simulink model "Consigna5_2_1"  (R2024b)
settings: Solver=ode45  StartTime=0.0  StopTime=20  RelTol=1e-3
values from neighbouring files (symbols this model uses):
  A_corrientes = [0 1; -omega_n_corrientes^2 -2*omega_n_corrientes]    [parametros.m]
  A_inversor = [0 1; -omega_n_inversor^2 -2*omega_n_inversor]    [parametros.m]
  A_posicion = [0 1; -omega_n_posicion^2 -2*omega_n_posicion]    [parametros.m]
  A_temp = -1/20    (= -0.05)    [parametros.m]
  alpha_cu = 3.9 *10^-3    (= 0.0039)    [parametros.m]
  B_corrientes = [0; omega_n_corrientes^2]    [parametros.m]
  b_eq = b_m + (1/r^2) * b_l    (= 2.19444444444e-05)    [parametros.m]
  B_inversor = [0; omega_n_inversor^2]    [parametros.m]
  b_l = 0.1    [parametros.m]
  b_m = 1.5 * 10^-5    (= 1.5e-05)    [parametros.m]
  B_posicion = [0; omega_n_posicion^2]    [parametros.m]
  B_temp = 1/20    (= 0.05)    [parametros.m]
  ba = J_eq*n*omega_pos    (= 0.0916527777778)    [parametros.m]
  C_corrientes = [1 0]    [parametros.m]
  C_inversor = [1 0]    [parametros.m]
  C_posicion = [1 0]    [parametros.m]
  C_temp = 1    [parametros.m]
  C_ts = 0.818    [parametros.m]
  g = 9.80665    [parametros.m]
  J_l = (m*l_cm^2 + J_cm) + (m_l * l_l^2)    (= 0.4583)    [parametros.m]
  J_m = 1.4 * 10^-5    (= 1.4e-05)    [parametros.m]
  K_e_int = 3200 ^3    (= 32768000000)    [parametros.m]
  K_e_omega = 3*3200^2    (= 30720000)    [parametros.m]
  K_e_theta = 9600    [parametros.m]
  k_l = m * l_cm + m_l* l_l    (= 1)    [parametros.m]
  Ksa = J_eq*n*(omega_pos^2)    (= 73.3222222222)    [parametros.m]
  Ksia = J_eq*(omega_pos^3)    (= 23463.1111111)    [parametros.m]
  L_d = 6.6 * 10^-3    (= 0.0066)    [parametros.m]
  L_ls = 0.8 * 10^-3    (= 0.0008)    [parametros.m]
  L_q = 5.8 * 10^-3    (= 0.0058)    [parametros.m]
  lambda_m = 0.016    [parametros.m]
  P_p = 3    [parametros.m]
  r = 120    [parametros.m]
  R_s_40 = 1.02    [parametros.m]
  R_ts_amb = 146.7    [parametros.m]
  T_sample = 1/f_sample    (= 4.53514739229e-05)    [parametros.m]
  Temp_s_ref = 20    [parametros.m]
  tm = X(1)    [parametros.m]
  tr = X(2)    [parametros.m]
  w2 = 188.49556    [parametros.m]
  x0_corrientes = [0;0]    [parametros.m]
  x0_inversor = [0;0]    [parametros.m]
  x0_posicion = [0; 0]    [parametros.m]
  x0_temp = 20    [parametros.m]
libraries: simulink x14, dspsigops x6
(part 2 of 4)

== system Consigna5_2_1/Subsystem1/Observador de estado reducido ==
  T_m* : Inport
  theta_m : Inport  Port=2
  Gain : Gain  Gain=1/(J_m+(J_l/r^2))
  Gain1 : Gain  Gain=K_e_theta
  Gain2 : Gain  Gain=K_e_omega
  Integrator : Integrator
  Integrator1 : Integrator
  Sum : Sum  Inputs=|++
  Sum1 : Sum  Inputs=|++
  Sum2 : Sum  Inputs=|-+
  omega_m_obs : Outport
  theta_m_obs : Outport  Port=2
  wires:
  T_m*/1 -> Gain/1
  Gain/1 -> Sum/1
  Sum/1 -> Integrator/1
  Integrator1/1 -> theta_m_obs/1, Sum2/1
  Integrator/1 -> Sum1/1
  Sum1/1 -> omega_m_obs/1, Integrator1/1
  theta_m/1 -> Sum2/2
  Gain1/1 -> Sum1/2
  Sum2/1 -> Gain2/1, Gain1/1
  Gain2/1 -> Sum/2

== system Consigna5_2_1/Subsystem1/Setpoint ==
  q1* : Inport
  Derivative : Derivative
  Gain : Gain  Gain=r
  theta_m* : Outport
  omega_m* : Outport  Port=2
  wires:
  q1*/1 -> Gain/1
  Gain/1 -> Derivative/1, theta_m*/1
  Derivative/1 -> omega_m*/1

== system Consigna5_2_1/Subsystem1/Subsistema físico no lineal ==
  note: Retroalimentación natural del torque gravitacional
  T_per : Inport
  v_as : Inport  Port=2
  v_bs : Inport  Port=3
  v_cs : Inport  Port=4
  Tº_amb : Inport  Port=5
  Gain : Gain  Gain=P_p
  Gain1 : Gain  Gain=1/r
  Gain2 : Gain  Gain=k_l
  Gain3 : Gain  Gain=g
  Mux : Mux  Inputs=3
  Scope : Scope
  Sin : Trigonometry
  Subsistema electromagnético : Subsystem
      settings: PortSchema="{\"entries\":[{\"content\":{\"sides\":[{\"content\":{\"connectorIds\":[\"In1\",\"In2\",\"In3\",\"In4\"]},\"type\":\"ConnectorPlacement.EquallySpacedRectSide\",\"uuid\":\"c9fae60f-a644-4c7d-9a50-e330e891aba8\"},{\"content\":{\"connectorIds\":[\"Out1\",\"Out2\",\"Out3\",\"Out4\"],\"side\":\"RIGHT\"},\"type\":\"ConnectorPlacement.EquallySpacedRectSide\",\"uuid\":\"1bd25713-f5e9-4106-83eb-fb9f8a30d88e\"},{\"content\":{\"connectorIds\":[\"In5\"],\"side\":\"TOP\"},\"type\":\"ConnectorPlacement.EquallySpacedRectSide\",\"uuid\":\"c2f005dd-e04f-426d-b804-ce475aa5422d\"}]},\"type\":\"ConnectorPlacement.EquallySpacedConnector\",\"uuid\":\"9bdc4406-fcef-47cb-a5c0-d4f33f547a91\"}],\"packageUris\":[\"http://schema.mathworks.com/mf0/Connector/R2020b\"],\"version\":\"1.0\"}"
  Subsistema mecánico completo : Subsystem
  Subsistema térmico : Subsystem
  Sum : Sum  Inputs=++|
  TD_PARK : MATLAB Function  TreatAsAtomicUnit=on
  TI_PARK : MATLAB Function  TreatAsAtomicUnit=on
  theta_m : Outport
  T_s : Outport  Port=2
  i_abcs : Outport  Port=3
  omega_m : Outport  Port=4
  T_m : Outport  Port=5
  T_l : Outport  Port=6
  wires:
  Subsistema electromagnético/4(T_m) -> T_m/1, Subsistema mecánico completo/1(T_m)
  Subsistema electromagnético/3(i_0s) -> Subsistema térmico/3(i_0s^r), TI_PARK/3(f0s)
  Subsistema mecánico completo/2(omega_m(t)) -> Subsistema electromagnético/5(omega_m), Scope/1, omega_m/1
  Subsistema electromagnético/1(i_qs^r) -> Subsistema térmico/1(i_qs^r), TI_PARK/1(fqs)
  Subsistema electromagnético/2(i_ds^r) -> Subsistema térmico/2(i_ds^r), TI_PARK/2(fds)
  Sum/1 -> T_l/1, Subsistema mecánico completo/2(T_l)  "T_l"
  TD_PARK/1(fqs) -> Subsistema electromagnético/1(v_qs^r)
  Tº_amb/1 -> Subsistema térmico/4(Tº_amb)
  Mux/1 -> i_abcs/1
  TI_PARK/1(fas) -> Mux/1
  TI_PARK/2(fbs) -> Mux/2
  TI_PARK/3(fcs) -> Mux/3
  v_as/1 -> TD_PARK/1(fas)
  v_cs/1 -> TD_PARK/3(fcs)
  Gain/1 -> TI_PARK/4(theta_r), TD_PARK/4(theta_r)
  v_bs/1 -> TD_PARK/2(fbs)
  Gain1/1 -> Sin/1
  Sin/1 -> Gain3/1
  Gain2/1 -> Sum/1
  T_per/1 -> Sum/2
  TD_PARK/2(fds) -> Subsistema electromagnético/2(v_ds^r)
  TD_PARK/3(f0s) -> Subsistema electromagnético/3(v_0s)
  Subsistema térmico/1(r_s) -> Subsistema electromagnético/4(r_s)
  Subsistema térmico/2(T_s) -> T_s/1
  Subsistema mecánico completo/1(theta_m(t)) -> theta_m/1, Gain1/1, Gain/1
  Gain3/1 -> Gain2/1

== system Consigna5_2_1/Subsystem2/Controlador PID ==
  note: ba: Proporcional al error de velocidad
  note: Ksa: Proporcional a la integral al error de velocidad
  note: Ksia: Porporcional a la doble Integral al error de velocidad
  omega_m* : Inport
  omega_m : Inport  Port=2
  Gain : Gain  Gain=ba
  Gain1 : Gain  Gain=Ksa
  Gain2 : Gain  Gain=Ksia
  Integrator : Integrator
  Integrator1 : Integrator
  Sum : Sum  Inputs=|+-
  Sum1 : Sum  Inputs=+++
  Tm* : Outport
  wires:
  omega_m*/1 -> Sum/1
  omega_m/1 -> Sum/2
  Sum/1 -> Integrator/1, Gain/1
  Integrator/1 -> Integrator1/1, Gain1/1
  Gain/1 -> Sum1/3
  Sum1/1 -> Tm*/1
  Gain1/1 -> Sum1/2
  Integrator1/1 -> Gain2/1
  Gain2/1 -> Sum1/1

== system Consigna5_2_1/Subsystem2/Inversor: Modulador de tensión ==
  v_as* : Inport
  v_bs* : Inport  Port=2
  v_cs* : Inport  Port=3
  Gain5 : Gain
  Gain6 : Gain
  Gain7 : Gain
  v_as : Outport
  v_bs : Outport  Port=2
  v_cs : Outport  Port=3
  wires:
  v_as*/1 -> Gain5/1
  Gain5/1 -> v_as/1
  v_cs*/1 -> Gain7/1
  v_bs*/1 -> Gain6/1
  Gain7/1 -> v_cs/1
  Gain6/1 -> v_bs/1

== system Consigna5_2_1/Subsystem2/MODULADOR DE TORQUE1 ==
  Tm* : Inport
  omega_m : Inport  Port=2
  i_qs^r : Inport  Port=3
  i_ds^r : Inport  Port=4
  i_0s : Inport  Port=5
  Ts : Inport  Port=6
  Calculo rs : Subsystem
  Constant5 : Constant  Value=0
  Desacoples Fisicos : Subsystem
  Lazo de Torque : Subsystem
  Modulador de corriente : Subsystem
  v_qs*' : Outport
  v_ds*' : Outport  Port=2
  v_0s*' : Outport  Port=3
  wires:
  Lazo de Torque/1(iqs*) -> Modulador de corriente/1(I_qs*)
  Modulador de corriente/3(v_0s*) -> Desacoples Fisicos/3(v_0s*)
  i_ds^r/1 -> Modulador de corriente/5(i_ds), Desacoples Fisicos/5(i_ds), Lazo de Torque/3(ids)
  Modulador de corriente/1(v_qs*) -> Desacoples Fisicos/1(v_qs*)
  Constant5/1 -> Modulador de corriente/2(I_ds*), Modulador de corriente/3(I_0s*)
  i_qs^r/1 -> Desacoples Fisicos/4(i_qs), Modulador de corriente/4(i_qs)
  Tm*/1 -> Lazo de Torque/1(Tm*)
  omega_m/1 -> Desacoples Fisicos/7(omega_m), Lazo de Torque/2(omega_m)
  Modulador de corriente/2(v_ds*) -> Desacoples Fisicos/2(v_ds*)
  i_0s/1 -> Desacoples Fisicos/6(i_0s), Modulador de corriente/6(i_0s)
  Desacoples Fisicos/2(v_ds*') -> v_ds*'/1
  Desacoples Fisicos/1(v_qs*') -> v_qs*'/1
  Desacoples Fisicos/3(v_0s*') -> v_0s*'/1
  Ts/1 -> Calculo rs/1(Ts)
  Calculo rs/1(r_s) -> Desacoples Fisicos/8(R_s)

== system Consigna5_2_1/Subsystem2/Observador de estado reducido ==
  T_m* : Inport
  theta_m : Inport  Port=2
  Gain : Gain  Gain=1/(J_m+(J_l/r^2))
  Gain1 : Gain  Gain=K_e_theta
  Gain2 : Gain  Gain=K_e_omega
  Integrator : Integrator
  Integrator1 : Integrator
  Sum : Sum  Inputs=|++
  Sum1 : Sum  Inputs=|++
  Sum2 : Sum  Inputs=|-+
  omega_m_obs : Outport
  theta_m_obs : Outport  Port=2
  wires:
  T_m*/1 -> Gain/1
  Gain/1 -> Sum/1
  Sum/1 -> Integrator/1
  Integrator1/1 -> theta_m_obs/1, Sum2/1
  Integrator/1 -> Sum1/1
  Sum1/1 -> omega_m_obs/1, Integrator1/1
  theta_m/1 -> Sum2/2
  Gain1/1 -> Sum1/2
  Sum2/1 -> Gain2/1, Gain1/1
  Gain2/1 -> Sum/2

== system Consigna5_2_1/Subsystem2/Setpoint ==
  q1* : Inport
  Derivative : Derivative
  Gain : Gain  Gain=r
  theta_m* : Outport
  omega_m* : Outport  Port=2
  wires:
  q1*/1 -> Gain/1
  Gain/1 -> Derivative/1, theta_m*/1
  Derivative/1 -> omega_m*/1

== system Consigna5_2_1/Subsystem2/Subsistema físico no lineal ==
  note: Retroalimentación natural del torque gravitacional
  T_per : Inport
  v_as : Inport  Port=2
  v_bs : Inport  Port=3
  v_cs : Inport  Port=4
  Tº_amb : Inport  Port=5
  Gain : Gain  Gain=P_p
  Gain1 : Gain  Gain=1/r
  Gain2 : Gain  Gain=k_l
  Gain3 : Gain  Gain=g
  Mux : Mux  Inputs=3
  Scope : Scope
  Sin : Trigonometry
  Subsistema electromagnético : Subsystem
      settings: PortSchema="{\"entries\":[{\"content\":{\"sides\":[{\"content\":{\"connectorIds\":[\"In1\",\"In2\",\"In3\",\"In4\"]},\"type\":\"ConnectorPlacement.EquallySpacedRectSide\",\"uuid\":\"c9fae60f-a644-4c7d-9a50-e330e891aba8\"},{\"content\":{\"connectorIds\":[\"Out1\",\"Out2\",\"Out3\",\"Out4\"],\"side\":\"RIGHT\"},\"type\":\"ConnectorPlacement.EquallySpacedRectSide\",\"uuid\":\"1bd25713-f5e9-4106-83eb-fb9f8a30d88e\"},{\"content\":{\"connectorIds\":[\"In5\"],\"side\":\"TOP\"},\"type\":\"ConnectorPlacement.EquallySpacedRectSide\",\"uuid\":\"c2f005dd-e04f-426d-b804-ce475aa5422d\"}]},\"type\":\"ConnectorPlacement.EquallySpacedConnector\",\"uuid\":\"9bdc4406-fcef-47cb-a5c0-d4f33f547a91\"}],\"packageUris\":[\"http://schema.mathworks.com/mf0/Connector/R2020b\"],\"version\":\"1.0\"}"
  Subsistema mecánico completo : Subsystem
  Subsistema térmico : Subsystem
  Sum : Sum  Inputs=++|
  TD_PARK : MATLAB Function  TreatAsAtomicUnit=on
  TI_PARK : MATLAB Function  TreatAsAtomicUnit=on
  theta_m : Outport
  T_s : Outport  Port=2
  i_abcs : Outport  Port=3
  omega_m : Outport  Port=4
  T_m : Outport  Port=5
  T_l : Outport  Port=6
  wires:
  Subsistema electromagnético/4(T_m) -> T_m/1, Subsistema mecánico completo/1(T_m)
  Subsistema electromagnético/3(i_0s) -> Subsistema térmico/3(i_0s^r), TI_PARK/3(f0s)
  Subsistema mecánico completo/2(omega_m(t)) -> Subsistema electromagnético/5(omega_m), Scope/1, omega_m/1
  Subsistema electromagnético/1(i_qs^r) -> Subsistema térmico/1(i_qs^r), TI_PARK/1(fqs)
  Subsistema electromagnético/2(i_ds^r) -> Subsistema térmico/2(i_ds^r), TI_PARK/2(fds)
  Sum/1 -> T_l/1, Subsistema mecánico completo/2(T_l)  "T_l"
  TD_PARK/1(fqs) -> Subsistema electromagnético/1(v_qs^r)
  Tº_amb/1 -> Subsistema térmico/4(Tº_amb)
  Mux/1 -> i_abcs/1
  TI_PARK/1(fas) -> Mux/1
  TI_PARK/2(fbs) -> Mux/2
  TI_PARK/3(fcs) -> Mux/3
  v_as/1 -> TD_PARK/1(fas)
  v_cs/1 -> TD_PARK/3(fcs)
  Gain/1 -> TI_PARK/4(theta_r), TD_PARK/4(theta_r)
  v_bs/1 -> TD_PARK/2(fbs)
  Gain1/1 -> Sin/1
  Sin/1 -> Gain3/1
  Gain2/1 -> Sum/1
  T_per/1 -> Sum/2
  TD_PARK/2(fds) -> Subsistema electromagnético/2(v_ds^r)
  TD_PARK/3(f0s) -> Subsistema electromagnético/3(v_0s)
  Subsistema térmico/1(r_s) -> Subsistema electromagnético/4(r_s)
  Subsistema térmico/2(T_s) -> T_s/1
  Subsistema mecánico completo/1(theta_m(t)) -> theta_m/1, Gain1/1, Gain/1
  Gain3/1 -> Gain2/1

== system Consigna5_2_1/Subsystem3/Controlador PID ==
  note: ba: Proporcional al error de velocidad
  note: Ksa: Proporcional a la integral al error de velocidad
  note: Ksia: Porporcional a la doble Integral al error de velocidad
  omega_m* : Inport
  omega_m : Inport  Port=2
  Gain : Gain  Gain=ba
  Gain1 : Gain  Gain=Ksa
  Gain2 : Gain  Gain=Ksia
  Integrator : Integrator
  Integrator1 : Integrator
  Sum : Sum  Inputs=|+-
  Sum1 : Sum  Inputs=+++
  Tm* : Outport
  wires:
  omega_m*/1 -> Sum/1
  omega_m/1 -> Sum/2
  Sum/1 -> Integrator/1, Gain/1
  Integrator/1 -> Integrator1/1, Gain1/1
  Gain/1 -> Sum1/3
  Sum1/1 -> Tm*/1
  Gain1/1 -> Sum1/2
  Integrator1/1 -> Gain2/1
  Gain2/1 -> Sum1/1

== system Consigna5_2_1/Subsystem3/Inversor: Modulador de tensión ==
  v_as* : Inport
  v_bs* : Inport  Port=2
  v_cs* : Inport  Port=3
  Gain5 : Gain
  Gain6 : Gain
  Gain7 : Gain
  v_as : Outport
  v_bs : Outport  Port=2
  v_cs : Outport  Port=3
  wires:
  v_as*/1 -> Gain5/1
  Gain5/1 -> v_as/1
  v_cs*/1 -> Gain7/1
  v_bs*/1 -> Gain6/1
  Gain7/1 -> v_cs/1
  Gain6/1 -> v_bs/1

== system Consigna5_2_1/Subsystem3/MODULADOR DE TORQUE1 ==
  Tm* : Inport
  omega_m : Inport  Port=2
  i_qs^r : Inport  Port=3
  i_ds^r : Inport  Port=4
  i_0s : Inport  Port=5
  Ts : Inport  Port=6
  Calculo rs : Subsystem
  Constant5 : Constant  Value=0
  Desacoples Fisicos : Subsystem
  Lazo de Torque : Subsystem
  Modulador de corriente : Subsystem
  v_qs*' : Outport
  v_ds*' : Outport  Port=2
  v_0s*' : Outport  Port=3
  wires:
  Lazo de Torque/1(iqs*) -> Modulador de corriente/1(I_qs*)
  Modulador de corriente/3(v_0s*) -> Desacoples Fisicos/3(v_0s*)
  i_ds^r/1 -> Modulador de corriente/5(i_ds), Desacoples Fisicos/5(i_ds), Lazo de Torque/3(ids)
  Modulador de corriente/1(v_qs*) -> Desacoples Fisicos/1(v_qs*)
  Constant5/1 -> Modulador de corriente/2(I_ds*), Modulador de corriente/3(I_0s*)
  i_qs^r/1 -> Desacoples Fisicos/4(i_qs), Modulador de corriente/4(i_qs)
  Tm*/1 -> Lazo de Torque/1(Tm*)
  omega_m/1 -> Desacoples Fisicos/7(omega_m), Lazo de Torque/2(omega_m)
  Modulador de corriente/2(v_ds*) -> Desacoples Fisicos/2(v_ds*)
  i_0s/1 -> Desacoples Fisicos/6(i_0s), Modulador de corriente/6(i_0s)
  Desacoples Fisicos/2(v_ds*') -> v_ds*'/1
  Desacoples Fisicos/1(v_qs*') -> v_qs*'/1
  Desacoples Fisicos/3(v_0s*') -> v_0s*'/1
  Ts/1 -> Calculo rs/1(Ts)
  Calculo rs/1(r_s) -> Desacoples Fisicos/8(R_s)

== system Consigna5_2_1/Subsystem3/Observador de estado mejorado ==
  T_m* : Inport
  theta_m : Inport  Port=2
  Gain : Gain  Gain=1/(J_m+(J_l/r^2))
  Gain1 : Gain  Gain=K_e_theta
  Gain2 : Gain  Gain=K_e_omega
  Gain3 : Gain  Gain=K_e_int
  Integrator : Integrator
  Integrator1 : Integrator
  Integrator2 : Integrator
  Sum : Sum  Inputs=|++
  Sum1 : Sum  Inputs=|++
  Sum2 : Sum  Inputs=|-+
  Sum3 : Sum  Inputs=|++
  omega_m_obs : Outport
  theta_m_obs : Outport  Port=2
  wires:
  theta_m/1 -> Sum2/2
  T_m*/1 -> Gain/1
  Integrator2/1 -> Sum3/2
  Sum/1 -> Integrator/1
  Integrator1/1 -> theta_m_obs/1, Sum2/1
  Gain3/1 -> Integrator2/1
  Gain2/1 -> Sum/2
  Integrator/1 -> Sum1/1
  Gain1/1 -> Sum1/2
  Sum1/1 -> omega_m_obs/1, Integrator1/1
  Gain/1 -> Sum3/1
  Sum3/1 -> Sum/1
  Sum2/1 -> Gain3/1, Gain2/1, Gain1/1

== system Consigna5_2_1/Subsystem3/Setpoint ==
  q1* : Inport
  Derivative : Derivative
  Gain : Gain  Gain=r
  theta_m* : Outport
  omega_m* : Outport  Port=2
  wires:
  q1*/1 -> Gain/1
  Gain/1 -> Derivative/1, theta_m*/1
  Derivative/1 -> omega_m*/1

== system Consigna5_2_1/Subsystem3/Subsistema físico no lineal ==
  note: Retroalimentación natural del torque gravitacional
  T_per : Inport
  v_as : Inport  Port=2
  v_bs : Inport  Port=3
  v_cs : Inport  Port=4
  Tº_amb : Inport  Port=5
  Gain : Gain  Gain=P_p
  Gain1 : Gain  Gain=1/r
  Gain2 : Gain  Gain=k_l
  Gain3 : Gain  Gain=g
  Mux : Mux  Inputs=3
  Scope : Scope
  Sin : Trigonometry
  Subsistema electromagnético : Subsystem
      settings: PortSchema="{\"entries\":[{\"content\":{\"sides\":[{\"content\":{\"connectorIds\":[\"In1\",\"In2\",\"In3\",\"In4\"]},\"type\":\"ConnectorPlacement.EquallySpacedRectSide\",\"uuid\":\"c9fae60f-a644-4c7d-9a50-e330e891aba8\"},{\"content\":{\"connectorIds\":[\"Out1\",\"Out2\",\"Out3\",\"Out4\"],\"side\":\"RIGHT\"},\"type\":\"ConnectorPlacement.EquallySpacedRectSide\",\"uuid\":\"1bd25713-f5e9-4106-83eb-fb9f8a30d88e\"},{\"content\":{\"connectorIds\":[\"In5\"],\"side\":\"TOP\"},\"type\":\"ConnectorPlacement.EquallySpacedRectSide\",\"uuid\":\"c2f005dd-e04f-426d-b804-ce475aa5422d\"}]},\"type\":\"ConnectorPlacement.EquallySpacedConnector\",\"uuid\":\"9bdc4406-fcef-47cb-a5c0-d4f33f547a91\"}],\"packageUris\":[\"http://schema.mathworks.com/mf0/Connector/R2020b\"],\"version\":\"1.0\"}"
  Subsistema mecánico completo : Subsystem
  Subsistema térmico : Subsystem
  Sum : Sum  Inputs=++|
  TD_PARK : MATLAB Function  TreatAsAtomicUnit=on
  TI_PARK : MATLAB Function  TreatAsAtomicUnit=on
  theta_m : Outport
  T_s : Outport  Port=2
  i_abcs : Outport  Port=3
  omega_m : Outport  Port=4
  T_m : Outport  Port=5
  T_l : Outport  Port=6
  wires:
  Subsistema electromagnético/4(T_m) -> T_m/1, Subsistema mecánico completo/1(T_m)
  Subsistema electromagnético/3(i_0s) -> Subsistema térmico/3(i_0s^r), TI_PARK/3(f0s)
  Subsistema mecánico completo/2(omega_m(t)) -> Subsistema electromagnético/5(omega_m), Scope/1, omega_m/1
  Subsistema electromagnético/1(i_qs^r) -> Subsistema térmico/1(i_qs^r), TI_PARK/1(fqs)
  Subsistema electromagnético/2(i_ds^r) -> Subsistema térmico/2(i_ds^r), TI_PARK/2(fds)
  Sum/1 -> T_l/1, Subsistema mecánico completo/2(T_l)  "T_l"
  TD_PARK/1(fqs) -> Subsistema electromagnético/1(v_qs^r)
  Tº_amb/1 -> Subsistema térmico/4(Tº_amb)
  Mux/1 -> i_abcs/1
  TI_PARK/1(fas) -> Mux/1
  TI_PARK/2(fbs) -> Mux/2
  TI_PARK/3(fcs) -> Mux/3
  v_as/1 -> TD_PARK/1(fas)
  v_cs/1 -> TD_PARK/3(fcs)
  Gain/1 -> TI_PARK/4(theta_r), TD_PARK/4(theta_r)
  v_bs/1 -> TD_PARK/2(fbs)
  Gain1/1 -> Sin/1
  Sin/1 -> Gain3/1
  Gain2/1 -> Sum/1
  T_per/1 -> Sum/2
  TD_PARK/2(fds) -> Subsistema electromagnético/2(v_ds^r)
  TD_PARK/3(f0s) -> Subsistema electromagnético/3(v_0s)
  Subsistema térmico/1(r_s) -> Subsistema electromagnético/4(r_s)
  Subsistema térmico/2(T_s) -> T_s/1
  Subsistema mecánico completo/1(theta_m(t)) -> theta_m/1, Gain1/1, Gain/1
  Gain3/1 -> Gain2/1

== system Consigna5_2_1/Subsystem4/Controlador PID ==
  note: ba: Proporcional al error de velocidad
  note: Ksa: Proporcional a la integral al error de velocidad
  note: Ksia: Porporcional a la doble Integral al error de velocidad
  omega_m* : Inport
  omega_m : Inport  Port=2
  Gain : Gain  Gain=ba
  Gain1 : Gain  Gain=Ksa
  Gain2 : Gain  Gain=Ksia
  Integrator : Integrator
  Integrator1 : Integrator
  Sum : Sum  Inputs=|+-
  Sum1 : Sum  Inputs=+++
  Tm* : Outport
  wires:
  omega_m*/1 -> Sum/1
  omega_m/1 -> Sum/2
  Sum/1 -> Integrator/1, Gain/1
  Integrator/1 -> Integrator1/1, Gain1/1
  Gain/1 -> Sum1/3
  Sum1/1 -> Tm*/1
  Gain1/1 -> Sum1/2
  Integrator1/1 -> Gain2/1
  Gain2/1 -> Sum1/1

== system Consigna5_2_1/Subsystem4/Inversor: Modulador de tensión ==
  v_as* : Inport
  v_bs* : Inport  Port=2
  v_cs* : Inport  Port=3
  Gain5 : Gain
  Gain6 : Gain
  Gain7 : Gain
  v_as : Outport
  v_bs : Outport  Port=2
  v_cs : Outport  Port=3
  wires:
  v_as*/1 -> Gain5/1
  Gain5/1 -> v_as/1
  v_cs*/1 -> Gain7/1
  v_bs*/1 -> Gain6/1
  Gain7/1 -> v_cs/1
  Gain6/1 -> v_bs/1

== system Consigna5_2_1/Subsystem4/MODULADOR DE TORQUE1 ==
  Tm* : Inport
  omega_m : Inport  Port=2
  i_qs^r : Inport  Port=3
  i_ds^r : Inport  Port=4
  i_0s : Inport  Port=5
  Ts : Inport  Port=6
  Calculo rs : Subsystem
  Constant5 : Constant  Value=0
  Desacoples Fisicos : Subsystem
  Lazo de Torque : Subsystem
  Modulador de corriente : Subsystem
  v_qs*' : Outport
  v_ds*' : Outport  Port=2
  v_0s*' : Outport  Port=3
  wires:
  Lazo de Torque/1(iqs*) -> Modulador de corriente/1(I_qs*)
  Modulador de corriente/3(v_0s*) -> Desacoples Fisicos/3(v_0s*)
  i_ds^r/1 -> Modulador de corriente/5(i_ds), Desacoples Fisicos/5(i_ds), Lazo de Torque/3(ids)
  Modulador de corriente/1(v_qs*) -> Desacoples Fisicos/1(v_qs*)
  Constant5/1 -> Modulador de corriente/2(I_ds*), Modulador de corriente/3(I_0s*)
  i_qs^r/1 -> Desacoples Fisicos/4(i_qs), Modulador de corriente/4(i_qs)
  Tm*/1 -> Lazo de Torque/1(Tm*)
  omega_m/1 -> Desacoples Fisicos/7(omega_m), Lazo de Torque/2(omega_m)
  Modulador de corriente/2(v_ds*) -> Desacoples Fisicos/2(v_ds*)
  i_0s/1 -> Desacoples Fisicos/6(i_0s), Modulador de corriente/6(i_0s)
  Desacoples Fisicos/2(v_ds*') -> v_ds*'/1
  Desacoples Fisicos/1(v_qs*') -> v_qs*'/1
  Desacoples Fisicos/3(v_0s*') -> v_0s*'/1
  Ts/1 -> Calculo rs/1(Ts)
  Calculo rs/1(r_s) -> Desacoples Fisicos/8(R_s)

== system Consigna5_2_1/Subsystem4/Observador de estado mejorado ==
  T_m* : Inport
  theta_m : Inport  Port=2
  Gain : Gain  Gain=1/(J_m+(J_l/r^2))
  Gain1 : Gain  Gain=K_e_theta
  Gain2 : Gain  Gain=K_e_omega
  Gain3 : Gain  Gain=K_e_int
  Integrator : Integrator
  Integrator1 : Integrator
  Integrator2 : Integrator
  Sum : Sum  Inputs=|++
  Sum1 : Sum  Inputs=|++
  Sum2 : Sum  Inputs=|-+
  Sum3 : Sum  Inputs=|++
  omega_m_obs : Outport
  theta_m_obs : Outport  Port=2
  wires:
  theta_m/1 -> Sum2/2
  T_m*/1 -> Gain/1
  Integrator2/1 -> Sum3/2
  Sum/1 -> Integrator/1
  Integrator1/1 -> theta_m_obs/1, Sum2/1
  Gain3/1 -> Integrator2/1
  Gain2/1 -> Sum/2
  Integrator/1 -> Sum1/1
  Gain1/1 -> Sum1/2
  Sum1/1 -> omega_m_obs/1, Integrator1/1
  Gain/1 -> Sum3/1
  Sum3/1 -> Sum/1
  Sum2/1 -> Gain3/1, Gain2/1, Gain1/1

== system Consigna5_2_1/Subsystem4/Setpoint ==
  q1* : Inport
  Derivative : Derivative
  Gain : Gain  Gain=r
  theta_m* : Outport
  omega_m* : Outport  Port=2
  wires:
  q1*/1 -> Gain/1
  Gain/1 -> Derivative/1, theta_m*/1
  Derivative/1 -> omega_m*/1

== system Consigna5_2_1/Subsystem4/Subsistema físico no lineal ==
  note: Retroalimentación natural del torque gravitacional
  T_per : Inport
  v_as : Inport  Port=2
  v_bs : Inport  Port=3
  v_cs : Inport  Port=4
  Tº_amb : Inport  Port=5
  Gain : Gain  Gain=P_p
  Gain1 : Gain  Gain=1/r
  Gain2 : Gain  Gain=k_l
  Gain3 : Gain  Gain=g
  Mux : Mux  Inputs=3
  Scope : Scope
  Sin : Trigonometry
  Subsistema electromagnético : Subsystem
      settings: PortSchema="{\"entries\":[{\"content\":{\"sides\":[{\"content\":{\"connectorIds\":[\"In1\",\"In2\",\"In3\",\"In4\"]},\"type\":\"ConnectorPlacement.EquallySpacedRectSide\",\"uuid\":\"c9fae60f-a644-4c7d-9a50-e330e891aba8\"},{\"content\":{\"connectorIds\":[\"Out1\",\"Out2\",\"Out3\",\"Out4\"],\"side\":\"RIGHT\"},\"type\":\"ConnectorPlacement.EquallySpacedRectSide\",\"uuid\":\"1bd25713-f5e9-4106-83eb-fb9f8a30d88e\"},{\"content\":{\"connectorIds\":[\"In5\"],\"side\":\"TOP\"},\"type\":\"ConnectorPlacement.EquallySpacedRectSide\",\"uuid\":\"c2f005dd-e04f-426d-b804-ce475aa5422d\"}]},\"type\":\"ConnectorPlacement.EquallySpacedConnector\",\"uuid\":\"9bdc4406-fcef-47cb-a5c0-d4f33f547a91\"}],\"packageUris\":[\"http://schema.mathworks.com/mf0/Connector/R2020b\"],\"version\":\"1.0\"}"
  Subsistema mecánico completo : Subsystem
  Subsistema térmico : Subsystem
  Sum : Sum  Inputs=++|
  TD_PARK : MATLAB Function  TreatAsAtomicUnit=on
  TI_PARK : MATLAB Function  TreatAsAtomicUnit=on
  theta_m : Outport
  T_s : Outport  Port=2
  i_abcs : Outport  Port=3
  omega_m : Outport  Port=4
  T_m : Outport  Port=5
  T_l : Outport  Port=6
  wires:
  Subsistema electromagnético/4(T_m) -> T_m/1, Subsistema mecánico completo/1(T_m)
  Subsistema electromagnético/3(i_0s) -> Subsistema térmico/3(i_0s^r), TI_PARK/3(f0s)
  Subsistema mecánico completo/2(omega_m(t)) -> Subsistema electromagnético/5(omega_m), Scope/1, omega_m/1
  Subsistema electromagnético/1(i_qs^r) -> Subsistema térmico/1(i_qs^r), TI_PARK/1(fqs)
  Subsistema electromagnético/2(i_ds^r) -> Subsistema térmico/2(i_ds^r), TI_PARK/2(fds)
  Sum/1 -> T_l/1, Subsistema mecánico completo/2(T_l)  "T_l"
  TD_PARK/1(fqs) -> Subsistema electromagnético/1(v_qs^r)
  Tº_amb/1 -> Subsistema térmico/4(Tº_amb)
  Mux/1 -> i_abcs/1
  TI_PARK/1(fas) -> Mux/1
  TI_PARK/2(fbs) -> Mux/2
  TI_PARK/3(fcs) -> Mux/3
  v_as/1 -> TD_PARK/1(fas)
  v_cs/1 -> TD_PARK/3(fcs)
  Gain/1 -> TI_PARK/4(theta_r), TD_PARK/4(theta_r)
  v_bs/1 -> TD_PARK/2(fbs)
  Gain1/1 -> Sin/1
  Sin/1 -> Gain3/1
  Gain2/1 -> Sum/1
  T_per/1 -> Sum/2
  TD_PARK/2(fds) -> Subsistema electromagnético/2(v_ds^r)
  TD_PARK/3(f0s) -> Subsistema electromagnético/3(v_0s)
  Subsistema térmico/1(r_s) -> Subsistema electromagnético/4(r_s)
  Subsistema térmico/2(T_s) -> T_s/1
  Subsistema mecánico completo/1(theta_m(t)) -> theta_m/1, Gain1/1, Gain/1
  Gain3/1 -> Gain2/1

== system Consigna5_2_1/Subsystem5/Controlador PID ==
  note: ba: Proporcional al error de velocidad
  note: Ksa: Proporcional a la integral al error de velocidad
  note: Ksia: Porporcional a la doble Integral al error de velocidad
  omega_m* : Inport
  omega_m : Inport  Port=2
  Gain : Gain  Gain=ba
  Gain1 : Gain  Gain=Ksa
  Gain2 : Gain  Gain=Ksia
  Integrator : Integrator
  Integrator1 : Integrator
  Sum : Sum  Inputs=|+-
  Sum1 : Sum  Inputs=+++
  Tm* : Outport
  wires:
  omega_m*/1 -> Sum/1
  omega_m/1 -> Sum/2
  Sum/1 -> Integrator/1, Gain/1
  Integrator/1 -> Integrator1/1, Gain1/1
  Gain/1 -> Sum1/3
  Sum1/1 -> Tm*/1
  Gain1/1 -> Sum1/2
  Integrator1/1 -> Gain2/1
  Gain2/1 -> Sum1/1

== system Consigna5_2_1/Subsystem5/Inversor: Modulador de tensión ==
  v_as* : Inport
  v_bs* : Inport  Port=2
  v_cs* : Inport  Port=3
  Gain5 : Gain
  Gain6 : Gain
  Gain7 : Gain
  v_as : Outport
  v_bs : Outport  Port=2
  v_cs : Outport  Port=3
  wires:
  v_as*/1 -> Gain5/1
  Gain5/1 -> v_as/1
  v_cs*/1 -> Gain7/1
  v_bs*/1 -> Gain6/1
  Gain7/1 -> v_cs/1
  Gain6/1 -> v_bs/1

== system Consigna5_2_1/Subsystem5/MODULADOR DE TORQUE1 ==
  Tm* : Inport
  omega_m : Inport  Port=2
  i_qs^r : Inport  Port=3
  i_ds^r : Inport  Port=4
  i_0s : Inport  Port=5
  Ts : Inport  Port=6
  Calculo rs : Subsystem
  Constant5 : Constant  Value=0
  Desacoples Fisicos : Subsystem
  Lazo de Torque : Subsystem
  Modulador de corriente : Subsystem
  v_qs*' : Outport
  v_ds*' : Outport  Port=2
  v_0s*' : Outport  Port=3
  wires:
  Lazo de Torque/1(iqs*) -> Modulador de corriente/1(I_qs*)
  Modulador de corriente/3(v_0s*) -> Desacoples Fisicos/3(v_0s*)
  i_ds^r/1 -> Modulador de corriente/5(i_ds), Desacoples Fisicos/5(i_ds), Lazo de Torque/3(ids)
  Modulador de corriente/1(v_qs*) -> Desacoples Fisicos/1(v_qs*)
  Constant5/1 -> Modulador de corriente/2(I_ds*), Modulador de corriente/3(I_0s*)
  i_qs^r/1 -> Desacoples Fisicos/4(i_qs), Modulador de corriente/4(i_qs)
  Tm*/1 -> Lazo de Torque/1(Tm*)
  omega_m/1 -> Desacoples Fisicos/7(omega_m), Lazo de Torque/2(omega_m)
  Modulador de corriente/2(v_ds*) -> Desacoples Fisicos/2(v_ds*)
  i_0s/1 -> Desacoples Fisicos/6(i_0s), Modulador de corriente/6(i_0s)
  Desacoples Fisicos/2(v_ds*') -> v_ds*'/1
  Desacoples Fisicos/1(v_qs*') -> v_qs*'/1
  Desacoples Fisicos/3(v_0s*') -> v_0s*'/1
  Ts/1 -> Calculo rs/1(Ts)
  Calculo rs/1(r_s) -> Desacoples Fisicos/8(R_s)

== system Consigna5_2_1/Subsystem5/Observador de estado mejorado ==
  T_m* : Inport
  theta_m : Inport  Port=2
  Gain : Gain  Gain=1/(J_m+(J_l/r^2))
  Gain1 : Gain  Gain=K_e_theta
  Gain2 : Gain  Gain=K_e_omega
  Gain3 : Gain  Gain=K_e_int
  Integrator : Integrator
  Integrator1 : Integrator
  Integrator2 : Integrator
  Sum : Sum  Inputs=|++
  Sum1 : Sum  Inputs=|++
  Sum2 : Sum  Inputs=|-+
  Sum3 : Sum  Inputs=|++
  omega_m_obs : Outport
  theta_m_obs : Outport  Port=2
  wires:
  theta_m/1 -> Sum2/2
  T_m*/1 -> Gain/1
  Integrator2/1 -> Sum3/2
  Sum/1 -> Integrator/1
  Integrator1/1 -> theta_m_obs/1, Sum2/1
  Gain3/1 -> Integrator2/1
  Gain2/1 -> Sum/2
  Integrator/1 -> Sum1/1
  Gain1/1 -> Sum1/2
  Sum1/1 -> omega_m_obs/1, Integrator1/1
  Gain/1 -> Sum3/1
  Sum3/1 -> Sum/1
  Sum2/1 -> Gain3/1, Gain2/1, Gain1/1

== system Consigna5_2_1/Subsystem5/Sensores ==
  theta_m : Inport
  T_s : Inport  Port=2
  i_as : Inport  Port=3
  i_bs : Inport  Port=4
  i_cs : Inport  Port=5
  S_corrientes : StateSpace  A=A_corrientes  B=B_corrientes  C=C_corrientes  D=0  InitialCondition=x0_corrientes
  S_corrientes1 : StateSpace  A=A_corrientes  B=B_corrientes  C=C_corrientes  D=0  InitialCondition=x0_corrientes
  S_corrientes2 : StateSpace  A=A_corrientes  B=B_corrientes  C=C_corrientes  D=0  InitialCondition=x0_corrientes
  S_posicion : StateSpace  A=A_posicion  B=B_posicion  C=C_posicion  D=0  InitialCondition=x0_posicion
  S_temp : StateSpace  A=A_temp  B=B_temp  C=C_temp  D=0  InitialCondition=x0_temp
  theta_m_medida : Outport
  T_s_medida : Outport  Port=2
  i_as_medida : Outport  Port=3
  i_bs_medida : Outport  Port=4
  i_cs_medida : Outport  Port=5
  wires:
  T_s/1 -> S_temp/1
  i_bs/1 -> S_corrientes1/1
  S_temp/1 -> T_s_medida/1
  i_as/1 -> S_corrientes/1
  i_cs/1 -> S_corrientes2/1
  S_corrientes/1 -> i_as_medida/1
  S_corrientes2/1 -> i_cs_medida/1
  S_corrientes1/1 -> i_bs_medida/1
  theta_m/1 -> S_posicion/1
  S_posicion/1 -> theta_m_medida/1

== system Consigna5_2_1/Subsystem5/Setpoint ==
  q1* : Inport
  Derivative : Derivative
  Gain : Gain  Gain=r
  theta_m* : Outport
  omega_m* : Outport  Port=2
  wires:
  q1*/1 -> Gain/1
  Gain/1 -> Derivative/1, theta_m*/1
  Derivative/1 -> omega_m*/1

== system Consigna5_2_1/Subsystem5/Subsistema físico no lineal ==
  note: Retroalimentación natural del torque gravitacional
  T_per : Inport
  v_as : Inport  Port=2
  v_bs : Inport  Port=3
  v_cs : Inport  Port=4
  Tº_amb : Inport  Port=5
  Gain : Gain  Gain=P_p
  Gain1 : Gain  Gain=1/r
  Gain2 : Gain  Gain=k_l
  Gain3 : Gain  Gain=g
  Mux : Mux  Inputs=3
  Scope : Scope
  Sin : Trigonometry
  Subsistema electromagnético : Subsystem
      settings: PortSchema="{\"entries\":[{\"content\":{\"sides\":[{\"content\":{\"connectorIds\":[\"In1\",\"In2\",\"In3\",\"In4\"]},\"type\":\"ConnectorPlacement.EquallySpacedRectSide\",\"uuid\":\"c9fae60f-a644-4c7d-9a50-e330e891aba8\"},{\"content\":{\"connectorIds\":[\"Out1\",\"Out2\",\"Out3\",\"Out4\"],\"side\":\"RIGHT\"},\"type\":\"ConnectorPlacement.EquallySpacedRectSide\",\"uuid\":\"1bd25713-f5e9-4106-83eb-fb9f8a30d88e\"},{\"content\":{\"connectorIds\":[\"In5\"],\"side\":\"TOP\"},\"type\":\"ConnectorPlacement.EquallySpacedRectSide\",\"uuid\":\"c2f005dd-e04f-426d-b804-ce475aa5422d\"}]},\"type\":\"ConnectorPlacement.EquallySpacedConnector\",\"uuid\":\"9bdc4406-fcef-47cb-a5c0-d4f33f547a91\"}],\"packageUris\":[\"http://schema.mathworks.com/mf0/Connector/R2020b\"],\"version\":\"1.0\"}"
  Subsistema mecánico completo : Subsystem
  Subsistema térmico : Subsystem
  Sum : Sum  Inputs=++|
  TD_PARK : MATLAB Function  TreatAsAtomicUnit=on
  TI_PARK : MATLAB Function  TreatAsAtomicUnit=on
  theta_m : Outport
  T_s : Outport  Port=2
  i_abcs : Outport  Port=3
  omega_m : Outport  Port=4
  T_m : Outport  Port=5
  T_l : Outport  Port=6
  wires:
  Subsistema electromagnético/4(T_m) -> T_m/1, Subsistema mecánico completo/1(T_m)
  Subsistema electromagnético/3(i_0s) -> Subsistema térmico/3(i_0s^r), TI_PARK/3(f0s)
  Subsistema mecánico completo/2(omega_m(t)) -> Subsistema electromagnético/5(omega_m), Scope/1, omega_m/1
  Subsistema electromagnético/1(i_qs^r) -> Subsistema térmico/1(i_qs^r), TI_PARK/1(fqs)
  Subsistema electromagnético/2(i_ds^r) -> Subsistema térmico/2(i_ds^r), TI_PARK/2(fds)
  Sum/1 -> T_l/1, Subsistema mecánico completo/2(T_l)  "T_l"
  TD_PARK/1(fqs) -> Subsistema electromagnético/1(v_qs^r)
  Tº_amb/1 -> Subsistema térmico/4(Tº_amb)
  Mux/1 -> i_abcs/1
  TI_PARK/1(fas) -> Mux/1
  TI_PARK/2(fbs) -> Mux/2
  TI_PARK/3(fcs) -> Mux/3
  v_as/1 -> TD_PARK/1(fas)
  v_cs/1 -> TD_PARK/3(fcs)
  Gain/1 -> TI_PARK/4(theta_r), TD_PARK/4(theta_r)
  v_bs/1 -> TD_PARK/2(fbs)
  Gain1/1 -> Sin/1
  Sin/1 -> Gain3/1
  Gain2/1 -> Sum/1
  T_per/1 -> Sum/2
  TD_PARK/2(fds) -> Subsistema electromagnético/2(v_ds^r)
  TD_PARK/3(f0s) -> Subsistema electromagnético/3(v_0s)
  Subsistema térmico/1(r_s) -> Subsistema electromagnético/4(r_s)
  Subsistema térmico/2(T_s) -> T_s/1
  Subsistema mecánico completo/1(theta_m(t)) -> theta_m/1, Gain1/1, Gain/1
  Gain3/1 -> Gain2/1

== system Consigna5_2_1/Subsystem6/CONTROLADOR PID ==
  note: ba: Proporcional al error de velocidad
  note: Ksa: Proporcional a la integral al error de velocidad
  note: Ksia: Porporcional a la doble Integral al error de velocidad
  omega_m* : Inport
  omega_m : Inport  Port=2
  Gain : Gain  Gain=ba
  Gain1 : Gain  Gain=Ksa
  Gain2 : Gain  Gain=Ksia
  Integrator : Integrator
  Integrator1 : Integrator
  Sum : Sum  Inputs=|+-
  Sum1 : Sum  Inputs=+++
  Tm* : Outport
  wires:
  omega_m*/1 -> Sum/1
  omega_m/1 -> Sum/2
  Sum/1 -> Integrator/1, Gain/1
  Integrator/1 -> Integrator1/1, Gain1/1
  Gain/1 -> Sum1/3
  Sum1/1 -> Tm*/1
  Gain1/1 -> Sum1/2
  Integrator1/1 -> Gain2/1
  Gain2/1 -> Sum1/1

== system Consigna5_2_1/Subsystem6/MODULADOR DE TORQUE1 ==
  Tm* : Inport
  omega_m : Inport  Port=2
  i_qs^r : Inport  Port=3
  i_ds^r : Inport  Port=4
  i_0s : Inport  Port=5
  Ts : Inport  Port=6
  Calculo rs : Subsystem
  Constant5 : Constant  Value=0
  Desacoples Fisicos : Subsystem
  Lazo de Torque : Subsystem
  Modulador de corriente : Subsystem
  v_qs*' : Outport
  v_ds*' : Outport  Port=2
  v_0s*' : Outport  Port=3
  wires:
  Lazo de Torque/1(iqs*) -> Modulador de corriente/1(I_qs*)
  Modulador de corriente/3(v_0s*) -> Desacoples Fisicos/3(v_0s*)
  i_ds^r/1 -> Modulador de corriente/5(i_ds), Desacoples Fisicos/5(i_ds), Lazo de Torque/3(ids)
  Modulador de corriente/1(v_qs*) -> Desacoples Fisicos/1(v_qs*)
  Constant5/1 -> Modulador de corriente/2(I_ds*), Modulador de corriente/3(I_0s*)
  i_qs^r/1 -> Desacoples Fisicos/4(i_qs), Modulador de corriente/4(i_qs)
  Tm*/1 -> Lazo de Torque/1(Tm*)
  omega_m/1 -> Desacoples Fisicos/7(omega_m), Lazo de Torque/2(omega_m)
  Modulador de corriente/2(v_ds*) -> Desacoples Fisicos/2(v_ds*)
  i_0s/1 -> Desacoples Fisicos/6(i_0s), Modulador de corriente/6(i_0s)
  Desacoples Fisicos/2(v_ds*') -> v_ds*'/1
  Desacoples Fisicos/1(v_qs*') -> v_qs*'/1
  Desacoples Fisicos/3(v_0s*') -> v_0s*'/1
  Ts/1 -> Calculo rs/1(Ts)
  Calculo rs/1(r_s) -> Desacoples Fisicos/8(R_s)

== system Consigna5_2_1/Subsystem6/MODULAR DE TENSIÓN NO IDEAL ==
  v_as* : Inport
  v_bs* : Inport  Port=2
  v_cs* : Inport  Port=3
  Saturation : Saturate  UpperLimit=39.192  LowerLimit=-39.192
  Saturation3 : Saturate  UpperLimit=39.192  LowerLimit=-39.192
  Saturation4 : Saturate  UpperLimit=39.192  LowerLimit=-39.192
  State-Space : StateSpace  A=A_inversor  B=B_inversor  C=C_inversor  InitialCondition=x0_inversor
  State-Space1 : StateSpace  A=A_inversor  B=B_inversor  C=C_inversor  InitialCondition=x0_inversor
  State-Space2 : StateSpace  A=A_inversor  B=B_inversor  C=C_inversor  InitialCondition=x0_inversor
  v_as : Outport
  v_bs : Outport  Port=2
  v_cs : Outport  Port=3
  wires:
  v_as*/1 -> State-Space/1
  State-Space/1 -> Saturation/1
  Saturation/1 -> v_as/1
  Saturation3/1 -> v_bs/1
  v_bs*/1 -> State-Space1/1
  State-Space1/1 -> Saturation3/1
  State-Space2/1 -> Saturation4/1
  Saturation4/1 -> v_cs/1
  v_cs*/1 -> State-Space2/1

== system Consigna5_2_1/Subsystem6/OBSERVADOR DE ESTADO MEJORADO ==
  T_m* : Inport
  theta_m : Inport  Port=2
  Gain : Gain  Gain=1/(J_m+(J_l/r^2))
  Gain1 : Gain  Gain=K_e_theta
  Gain2 : Gain  Gain=K_e_omega
  Gain3 : Gain  Gain=K_e_int
  Integrator : Integrator
  Integrator1 : Integrator
  Integrator2 : Integrator
  Sum : Sum  Inputs=|++
  Sum1 : Sum  Inputs=|++
  Sum2 : Sum  Inputs=|-+
  Sum3 : Sum  Inputs=|++
  omega_m_obs : Outport
  theta_m_obs : Outport  Port=2
  wires:
  theta_m/1 -> Sum2/2
  T_m*/1 -> Gain/1
  Integrator2/1 -> Sum3/2
  Sum/1 -> Integrator/1
  Integrator1/1 -> theta_m_obs/1, Sum2/1
  Gain3/1 -> Integrator2/1
  Gain2/1 -> Sum/2
  Integrator/1 -> Sum1/1
  Gain1/1 -> Sum1/2
  Sum1/1 -> omega_m_obs/1, Integrator1/1
  Gain/1 -> Sum3/1
  Sum3/1 -> Sum/1
  Sum2/1 -> Gain3/1, Gain2/1, Gain1/1

== system Consigna5_2_1/Subsystem6/PLANTA ==
  note: Retroalimentación natural del torque gravitacional
  T_per : Inport
  v_as : Inport  Port=2
  v_bs : Inport  Port=3
  v_cs : Inport  Port=4
  Tº_amb : Inport  Port=5
  Gain : Gain  Gain=P_p
  Gain1 : Gain  Gain=1/r
  Gain2 : Gain  Gain=k_l
  Gain3 : Gain  Gain=g
  Mux : Mux  Inputs=3
  Scope : Scope
  Sin : Trigonometry
  Subsistema electromagnético : Subsystem
      settings: PortSchema="{\"entries\":[{\"content\":{\"sides\":[{\"content\":{\"connectorIds\":[\"In1\",\"In2\",\"In3\",\"In4\"]},\"type\":\"ConnectorPlacement.EquallySpacedRectSide\",\"uuid\":\"c9fae60f-a644-4c7d-9a50-e330e891aba8\"},{\"content\":{\"connectorIds\":[\"Out1\",\"Out2\",\"Out3\",\"Out4\"],\"side\":\"RIGHT\"},\"type\":\"ConnectorPlacement.EquallySpacedRectSide\",\"uuid\":\"1bd25713-f5e9-4106-83eb-fb9f8a30d88e\"},{\"content\":{\"connectorIds\":[\"In5\"],\"side\":\"TOP\"},\"type\":\"ConnectorPlacement.EquallySpacedRectSide\",\"uuid\":\"c2f005dd-e04f-426d-b804-ce475aa5422d\"}]},\"type\":\"ConnectorPlacement.EquallySpacedConnector\",\"uuid\":\"9bdc4406-fcef-47cb-a5c0-d4f33f547a91\"}],\"packageUris\":[\"http://schema.mathworks.com/mf0/Connector/R2020b\"],\"version\":\"1.0\"}"
  Subsistema mecánico completo : Subsystem
  Subsistema térmico : Subsystem
  Sum : Sum  Inputs=++|
  TD_PARK : MATLAB Function  TreatAsAtomicUnit=on
  TI_PARK : MATLAB Function  TreatAsAtomicUnit=on
  theta_m : Outport
  T_s : Outport  Port=2
  i_abcs : Outport  Port=3
  omega_m : Outport  Port=4
  T_m : Outport  Port=5
  T_l : Outport  Port=6
  wires:
  Subsistema electromagnético/4(T_m) -> T_m/1, Subsistema mecánico completo/1(T_m)
  Subsistema electromagnético/3(i_0s) -> Subsistema térmico/3(i_0s^r), TI_PARK/3(f0s)
  Subsistema mecánico completo/2(omega_m(t)) -> Subsistema electromagnético/5(omega_m), Scope/1, omega_m/1
  Subsistema electromagnético/1(i_qs^r) -> Subsistema térmico/1(i_qs^r), TI_PARK/1(fqs)
  Subsistema electromagnético/2(i_ds^r) -> Subsistema térmico/2(i_ds^r), TI_PARK/2(fds)
  Sum/1 -> T_l/1, Subsistema mecánico completo/2(T_l)  "T_l"
  TD_PARK/1(fqs) -> Subsistema electromagnético/1(v_qs^r)
  Tº_amb/1 -> Subsistema térmico/4(Tº_amb)
  Mux/1 -> i_abcs/1
  TI_PARK/1(fas) -> Mux/1
  TI_PARK/2(fbs) -> Mux/2
  TI_PARK/3(fcs) -> Mux/3
  v_as/1 -> TD_PARK/1(fas)
  v_cs/1 -> TD_PARK/3(fcs)
  Gain/1 -> TI_PARK/4(theta_r), TD_PARK/4(theta_r)
  v_bs/1 -> TD_PARK/2(fbs)
  Gain1/1 -> Sin/1
  Sin/1 -> Gain3/1
  Gain2/1 -> Sum/1
  T_per/1 -> Sum/2
  TD_PARK/2(fds) -> Subsistema electromagnético/2(v_ds^r)
  TD_PARK/3(f0s) -> Subsistema electromagnético/3(v_0s)
  Subsistema térmico/1(r_s) -> Subsistema electromagnético/4(r_s)
  Subsistema térmico/2(T_s) -> T_s/1
  Subsistema mecánico completo/1(theta_m(t)) -> theta_m/1, Gain1/1, Gain/1
  Gain3/1 -> Gain2/1

== system Consigna5_2_1/Subsystem6/SENSORES NO IDEALES ==
  theta_m : Inport
  T_s : Inport  Port=2
  i_as : Inport  Port=3
  i_bs : Inport  Port=4
  i_cs : Inport  Port=5
  S_corrientes : StateSpace  A=A_corrientes  B=B_corrientes  C=C_corrientes  D=0  InitialCondition=x0_corrientes
  S_corrientes1 : StateSpace  A=A_corrientes  B=B_corrientes  C=C_corrientes  D=0  InitialCondition=x0_corrientes
  S_corrientes2 : StateSpace  A=A_corrientes  B=B_corrientes  C=C_corrientes  D=0  InitialCondition=x0_corrientes
  S_posicion : StateSpace  A=A_posicion  B=B_posicion  C=C_posicion  D=0  InitialCondition=x0_posicion
  S_temp : StateSpace  A=A_temp  B=B_temp  C=C_temp  D=0  InitialCondition=x0_temp
  theta_m_medida : Outport
  T_s_medida : Outport  Port=2
  i_as_medida : Outport  Port=3
  i_bs_medida : Outport  Port=4
  i_cs_medida : Outport  Port=5
  wires:
  T_s/1 -> S_temp/1
  i_bs/1 -> S_corrientes1/1
  S_temp/1 -> T_s_medida/1
  i_as/1 -> S_corrientes/1
  i_cs/1 -> S_corrientes2/1
  S_corrientes/1 -> i_as_medida/1
  S_corrientes2/1 -> i_cs_medida/1
  S_corrientes1/1 -> i_bs_medida/1
  theta_m/1 -> S_posicion/1
  S_posicion/1 -> theta_m_medida/1

== system Consigna5_2_1/Subsystem6/SETPOINT ==
  q1* : Inport
  Derivative : Derivative
  Gain : Gain  Gain=r
  theta_m* : Outport
  omega_m* : Outport  Port=2
  wires:
  q1*/1 -> Gain/1
  Gain/1 -> Derivative/1, theta_m*/1
  Derivative/1 -> omega_m*/1

== system Consigna5_2_1/Subsystem7/CONTROLADOR PID ==
  note: ba: Proporcional al error de velocidad
  note: Ksa: Proporcional a la integral al error de velocidad
  note: Ksia: Porporcional a la doble Integral al error de velocidad
  omega_m* : Inport
  omega_m : Inport  Port=2
  Gain : Gain  Gain=ba
  Gain1 : Gain  Gain=Ksa
  Gain2 : Gain  Gain=Ksia
  Integrator : Integrator
  Integrator1 : Integrator
  Sum : Sum  Inputs=|+-
  Sum1 : Sum  Inputs=+++
  Tm* : Outport
  wires:
  omega_m*/1 -> Sum/1
  omega_m/1 -> Sum/2
  Sum/1 -> Integrator/1, Gain/1
  Integrator/1 -> Integrator1/1, Gain1/1
  Gain/1 -> Sum1/3
  Sum1/1 -> Tm*/1
  Gain1/1 -> Sum1/2
  Integrator1/1 -> Gain2/1
  Gain2/1 -> Sum1/1

== system Consigna5_2_1/Subsystem7/MODULADOR DE TORQUE1 ==
  Tm* : Inport
  omega_m : Inport  Port=2
  i_qs^r : Inport  Port=3
  i_ds^r : Inport  Port=4
  i_0s : Inport  Port=5
  Ts : Inport  Port=6
  Calculo rs : Subsystem
  Constant5 : Constant  Value=0
  Desacoples Fisicos : Subsystem
  Lazo de Torque : Subsystem
  Modulador de corriente : Subsystem
  v_qs*' : Outport
  v_ds*' : Outport  Port=2
  v_0s*' : Outport  Port=3
  wires:
  Lazo de Torque/1(iqs*) -> Modulador de corriente/1(I_qs*)
  Modulador de corriente/3(v_0s*) -> Desacoples Fisicos/3(v_0s*)
  i_ds^r/1 -> Modulador de corriente/5(i_ds), Desacoples Fisicos/5(i_ds), Lazo de Torque/3(ids)
  Modulador de corriente/1(v_qs*) -> Desacoples Fisicos/1(v_qs*)
  Constant5/1 -> Modulador de corriente/2(I_ds*), Modulador de corriente/3(I_0s*)
  i_qs^r/1 -> Desacoples Fisicos/4(i_qs), Modulador de corriente/4(i_qs)
  Tm*/1 -> Lazo de Torque/1(Tm*)
  omega_m/1 -> Desacoples Fisicos/7(omega_m), Lazo de Torque/2(omega_m)
  Modulador de corriente/2(v_ds*) -> Desacoples Fisicos/2(v_ds*)
  i_0s/1 -> Desacoples Fisicos/6(i_0s), Modulador de corriente/6(i_0s)
  Desacoples Fisicos/2(v_ds*') -> v_ds*'/1
  Desacoples Fisicos/1(v_qs*') -> v_qs*'/1
  Desacoples Fisicos/3(v_0s*') -> v_0s*'/1
  Ts/1 -> Calculo rs/1(Ts)
  Calculo rs/1(r_s) -> Desacoples Fisicos/8(R_s)

== system Consigna5_2_1/Subsystem7/MODULAR DE TENSIÓN NO IDEAL ==
  v_as* : Inport
  v_bs* : Inport  Port=2
  v_cs* : Inport  Port=3
  Saturation : Saturate  UpperLimit=39.192  LowerLimit=-39.192
  Saturation3 : Saturate  UpperLimit=39.192  LowerLimit=-39.192
  Saturation4 : Saturate  UpperLimit=39.192  LowerLimit=-39.192
  State-Space : StateSpace  A=A_inversor  B=B_inversor  C=C_inversor  InitialCondition=x0_inversor
  State-Space1 : StateSpace  A=A_inversor  B=B_inversor  C=C_inversor  InitialCondition=x0_inversor
  State-Space2 : StateSpace  A=A_inversor  B=B_inversor  C=C_inversor  InitialCondition=x0_inversor
  v_as : Outport
  v_bs : Outport  Port=2
  v_cs : Outport  Port=3
  wires:
  v_as*/1 -> State-Space/1
  State-Space/1 -> Saturation/1
  Saturation/1 -> v_as/1
  Saturation3/1 -> v_bs/1
  v_bs*/1 -> State-Space1/1
  State-Space1/1 -> Saturation3/1
  State-Space2/1 -> Saturation4/1
  Saturation4/1 -> v_cs/1
  v_cs*/1 -> State-Space2/1

== system Consigna5_2_1/Subsystem7/OBSERVADOR DE ESTADO MEJORADO ==
  T_m* : Inport
  theta_m : Inport  Port=2
  Gain : Gain  Gain=1/(J_m+(J_l/r^2))
  Gain1 : Gain  Gain=K_e_theta
  Gain2 : Gain  Gain=K_e_omega
  Gain3 : Gain  Gain=K_e_int
  Integrator : Integrator
  Integrator1 : Integrator
  Integrator2 : Integrator
  Sum : Sum  Inputs=|++
  Sum1 : Sum  Inputs=|++
  Sum2 : Sum  Inputs=|-+
  Sum3 : Sum  Inputs=|++
  omega_m_obs : Outport
  theta_m_obs : Outport  Port=2
  wires:
  theta_m/1 -> Sum2/2
  T_m*/1 -> Gain/1
  Integrator2/1 -> Sum3/2
  Sum/1 -> Integrator/1
  Integrator1/1 -> theta_m_obs/1, Sum2/1
  Gain3/1 -> Integrator2/1
  Gain2/1 -> Sum/2
  Integrator/1 -> Sum1/1
  Gain1/1 -> Sum1/2
  Sum1/1 -> omega_m_obs/1, Integrator1/1
  Gain/1 -> Sum3/1
  Sum3/1 -> Sum/1
  Sum2/1 -> Gain3/1, Gain2/1, Gain1/1

== system Consigna5_2_1/Subsystem7/PLANTA ==
  note: Retroalimentación natural del torque gravitacional
  T_per : Inport
  v_as : Inport  Port=2
  v_bs : Inport  Port=3
  v_cs : Inport  Port=4
  Tº_amb : Inport  Port=5
  Gain : Gain  Gain=P_p
  Gain1 : Gain  Gain=1/r
  Gain2 : Gain  Gain=k_l
  Gain3 : Gain  Gain=g
  Mux : Mux  Inputs=3
  Scope : Scope
  Sin : Trigonometry
  Subsistema electromagnético : Subsystem
      settings: PortSchema="{\"entries\":[{\"content\":{\"sides\":[{\"content\":{\"connectorIds\":[\"In1\",\"In2\",\"In3\",\"In4\"]},\"type\":\"ConnectorPlacement.EquallySpacedRectSide\",\"uuid\":\"c9fae60f-a644-4c7d-9a50-e330e891aba8\"},{\"content\":{\"connectorIds\":[\"Out1\",\"Out2\",\"Out3\",\"Out4\"],\"side\":\"RIGHT\"},\"type\":\"ConnectorPlacement.EquallySpacedRectSide\",\"uuid\":\"1bd25713-f5e9-4106-83eb-fb9f8a30d88e\"},{\"content\":{\"connectorIds\":[\"In5\"],\"side\":\"TOP\"},\"type\":\"ConnectorPlacement.EquallySpacedRectSide\",\"uuid\":\"c2f005dd-e04f-426d-b804-ce475aa5422d\"}]},\"type\":\"ConnectorPlacement.EquallySpacedConnector\",\"uuid\":\"9bdc4406-fcef-47cb-a5c0-d4f33f547a91\"}],\"packageUris\":[\"http://schema.mathworks.com/mf0/Connector/R2020b\"],\"version\":\"1.0\"}"
  Subsistema mecánico completo : Subsystem
  Subsistema térmico : Subsystem
  Sum : Sum  Inputs=++|
  TD_PARK : MATLAB Function  TreatAsAtomicUnit=on
  TI_PARK : MATLAB Function  TreatAsAtomicUnit=on
  theta_m : Outport
  T_s : Outport  Port=2
  i_abcs : Outport  Port=3
  omega_m : Outport  Port=4
  T_m : Outport  Port=5
  T_l : Outport  Port=6
  wires:
  Subsistema electromagnético/4(T_m) -> T_m/1, Subsistema mecánico completo/1(T_m)
  Subsistema electromagnético/3(i_0s) -> Subsistema térmico/3(i_0s^r), TI_PARK/3(f0s)
  Subsistema mecánico completo/2(omega_m(t)) -> Subsistema electromagnético/5(omega_m), Scope/1, omega_m/1
  Subsistema electromagnético/1(i_qs^r) -> Subsistema térmico/1(i_qs^r), TI_PARK/1(fqs)
  Subsistema electromagnético/2(i_ds^r) -> Subsistema térmico/2(i_ds^r), TI_PARK/2(fds)
  Sum/1 -> T_l/1, Subsistema mecánico completo/2(T_l)  "T_l"
  TD_PARK/1(fqs) -> Subsistema electromagnético/1(v_qs^r)
  Tº_amb/1 -> Subsistema térmico/4(Tº_amb)
  Mux/1 -> i_abcs/1
  TI_PARK/1(fas) -> Mux/1
  TI_PARK/2(fbs) -> Mux/2
  TI_PARK/3(fcs) -> Mux/3
  v_as/1 -> TD_PARK/1(fas)
  v_cs/1 -> TD_PARK/3(fcs)
  Gain/1 -> TI_PARK/4(theta_r), TD_PARK/4(theta_r)
  v_bs/1 -> TD_PARK/2(fbs)
  Gain1/1 -> Sin/1
  Sin/1 -> Gain3/1
  Gain2/1 -> Sum/1
  T_per/1 -> Sum/2
  TD_PARK/2(fds) -> Subsistema electromagnético/2(v_ds^r)
  TD_PARK/3(f0s) -> Subsistema electromagnético/3(v_0s)
  Subsistema térmico/1(r_s) -> Subsistema electromagnético/4(r_s)
  Subsistema térmico/2(T_s) -> T_s/1
  Subsistema mecánico completo/1(theta_m(t)) -> theta_m/1, Gain1/1, Gain/1
  Gain3/1 -> Gain2/1

== system Consigna5_2_1/Subsystem7/S&H X3 ==
  u1 : Inport
  u2 : Inport  Port=2
  u3 : Inport  Port=3
  Pulse Generator1 : DiscretePulseGenerator  PulseType=Time based  Period=T_sample  PulseWidth=50
  Pulse Generator2 : DiscretePulseGenerator  PulseType=Time based  Period=T_sample  PulseWidth=50
  Pulse Generator3 : DiscretePulseGenerator  PulseType=Time based  Period=T_sample  PulseWidth=50
  Sample and Hold1 : dspsigops/Sample and Hold  trig=Rising edge  initCond=0  latchinput=off
  Sample and Hold2 : dspsigops/Sample and Hold  trig=Rising edge  initCond=0  latchinput=off
  Sample and Hold3 : dspsigops/Sample and Hold  trig=Rising edge  initCond=0  latchinput=off
  y1 : Outport
  y2 : Outport  Port=2
  y3 : Outport  Port=3
  wires:
  u1/1 -> Sample and Hold2/1
  Pulse Generator2/1 -> Sample and Hold2/Trigger
  Sample and Hold2/1 -> y1/1  "y discreta"
  Sample and Hold1/1 -> y2/1  "y discreta"
  u2/1 -> Sample and Hold1/1
  Pulse Generator1/1 -> Sample and Hold1/Trigger
  Sample and Hold3/1 -> y3/1  "y discreta"
  Pulse Generator3/1 -> Sample and Hold3/Trigger
  u3/1 -> Sample and Hold3/1

== system Consigna5_2_1/Subsystem7/SENSORES NO IDEALES ==
  theta_m : Inport
  T_s : Inport  Port=2
  i_as : Inport  Port=3
  i_bs : Inport  Port=4
  i_cs : Inport  Port=5
  S_corrientes : StateSpace  A=A_corrientes  B=B_corrientes  C=C_corrientes  D=0  InitialCondition=x0_corrientes
  S_corrientes1 : StateSpace  A=A_corrientes  B=B_corrientes  C=C_corrientes  D=0  InitialCondition=x0_corrientes
  S_corrientes2 : StateSpace  A=A_corrientes  B=B_corrientes  C=C_corrientes  D=0  InitialCondition=x0_corrientes
  S_posicion : StateSpace  A=A_posicion  B=B_posicion  C=C_posicion  D=0  InitialCondition=x0_posicion
  S_temp : StateSpace  A=A_temp  B=B_temp  C=C_temp  D=0  InitialCondition=x0_temp
  theta_m_medida : Outport
  T_s_medida : Outport  Port=2
  i_as_medida : Outport  Port=3
  i_bs_medida : Outport  Port=4
  i_cs_medida : Outport  Port=5
  wires:
  T_s/1 -> S_temp/1
  i_bs/1 -> S_corrientes1/1
  S_temp/1 -> T_s_medida/1
  i_as/1 -> S_corrientes/1
  i_cs/1 -> S_corrientes2/1
  S_corrientes/1 -> i_as_medida/1
  S_corrientes2/1 -> i_cs_medida/1
  S_corrientes1/1 -> i_bs_medida/1
  theta_m/1 -> S_posicion/1
  S_posicion/1 -> theta_m_medida/1

== system Consigna5_2_1/Subsystem7/SETPOINT ==
  q1* : Inport
  Derivative : Derivative
  Gain : Gain  Gain=r
  theta_m* : Outport
  omega_m* : Outport  Port=2
  wires:
  q1*/1 -> Gain/1
  Gain/1 -> Derivative/1, theta_m*/1
  Derivative/1 -> omega_m*/1
